simulink library "colorDetector"  (R2018b)
settings: Solver=VariableStepAuto  StartTime=0.0  StopTime=10.0  RelTol=1e-3
settings Model: Creator=anna  LastModifiedBy=Sjoerd

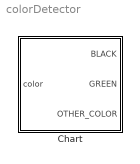
== system colorDetector ==
  Chart : Stateflow chart  TreatAsAtomicUnit=on

== stateflow chart colorDetector/Chart ==
  state otherColor
    entry:
    OTHER_COLOR = true
    exit:
    OTHER_COLOR = false
  state blackColor
    entry:
    BLACK = true
    exit:
    BLACK = false
  state greenColor
    entry:
    GREEN = true
    exit:
    GREEN = false
  (default) -> otherColor
  otherColor -> blackColor [order 1] : [color==1]
  blackColor -> otherColor [order 1] : [color~=1&& color~=3]
  greenColor -> blackColor [order 2] : [color==1]
  blackColor -> greenColor [order 2] : [color==3]
  greenColor -> otherColor [order 1] : [color~=1&& color~=3]
  otherColor -> greenColor [order 2] : [color==3]
  data: color input; BLACK output boolean size=1; GREEN output boolean size=1; OTHER_COLOR output boolean size=1
